simulink model "CTRL_LO_ST1_YAWTRQLGT_test"  (R2023b)
settings: Solver=VariableStepAuto  StartTime=0.0  StopTime=10.0  RelTol=1e-3
libraries: CTRL_LO_ST1_YAWTRQLGT x1
settings Model: Creator=blatak  LastModifiedBy=blatak

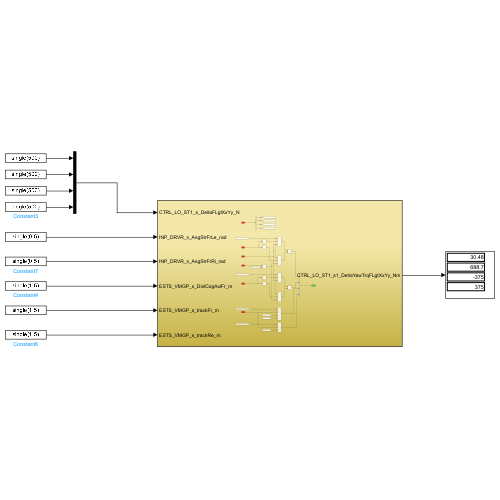
[thumbnail: Simulink's stored preview of the top-level diagram]
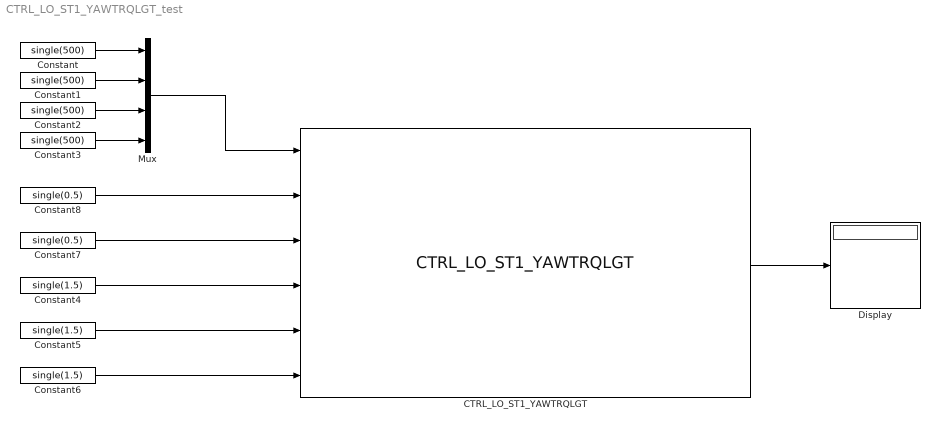
== system CTRL_LO_ST1_YAWTRQLGT_test ==
  CTRL_LO_ST1_YAWTRQLGT : CTRL_LO_ST1_YAWTRQLGT/CTRL_LO_ST1_YAWTRQLGT  SystemSampleTime=-1  VariantActivationTime=update diagram  AllowFlexibleInterface=on  Latency=0  AutoFrameSizeCalculation=off
  Constant{,1..3} (4 alike) : Constant  Value=single(500)
  Constant4 : Constant  Value=single(1.5)
  Constant5 : Constant  Value=single(1.5)
  Constant6 : Constant  Value=single(1.5)
  Constant7 : Constant  Value=single(0.5)
  Constant8 : Constant  Value=single(0.5)
  Display : Display
  Mux : Mux
  wires:
  Constant/1 -> Mux/1
  Constant1/1 -> Mux/2
  Constant2/1 -> Mux/3
  Constant3/1 -> Mux/4
  Mux/1 -> CTRL_LO_ST1_YAWTRQLGT/1
  Constant4/1 -> CTRL_LO_ST1_YAWTRQLGT/4
  Constant6/1 -> CTRL_LO_ST1_YAWTRQLGT/6
  Constant5/1 -> CTRL_LO_ST1_YAWTRQLGT/5
  Constant7/1 -> CTRL_LO_ST1_YAWTRQLGT/3
  Constant8/1 -> CTRL_LO_ST1_YAWTRQLGT/2
  CTRL_LO_ST1_YAWTRQLGT/1 -> Display/1
